simulink model "EvPowertrainController3EMDualRear"  (R2024a)
settings: configuration reference "VehicleFixed10ms" (kept outside this file)
model workspace (MAT data in the model file):
  CtrlVcuAccelPdlBpts = [0 0.8 1]
  CtrlVcuBattPnlty = 10000000
  CtrlVcuBattSOCBpts = [0 20 60 80 100]
  CtrlVcuCnstrntPnltyFctr = 10000000
  CtrlVcuEMPnlty = 100
  CtrlVcuEMTrqSplitGrid = 200
  CtrlVcuFallRate = -500
  CtrlVcuMaxAccelG = 1
  CtrlVcuMaxDecelG = -1.5
  CtrlVcuPwrDeltaPnlty = 50
  CtrlVcuPwrRatePnlty = [25 25 100]
  CtrlVcuRiseRate = 500
  CtrlVcuRoadMuEst = 0.8
  CtrlVcuSftyFctr = 0.9
  CtrlVcuTracPwrErrPnlty = 25
  CtrlVcuTrqVecBrkThresh = 0.01
  CtrlVcuTrqVecIGain = 0
  CtrlVcuTrqVecMinTrq = 25
  CtrlVcuTrqVecPGain = -2000
  CtrlVcuTrqVecSteerThresh = 0.349065850399
  CtrlVcuTrqVecVelThresh = 2.5
  N_P0 = 3
undefined symbols (not defined in the file): CtrlBcuTrlrBrkGain, CtrlVcuEvChrgLmtBpt, CtrlVcuEvRegenBrkCutOff, CtrlVcuEvRegenBrkSpdBpt, CtrlVcuEvSocBpt, eff, EnvGrvty, PlntBrkActrBoreFrnt, PlntBrkFrntBias, PlntBrkKinFricCffFrnt, PlntBrkNumPadsFrnt, PlntBrkPadMeanRadiusFrnt, PlntBrkPrsFctr, PlntBrkRearBias, PlntDiffrntl2Eff, PlntDiffrntl2Ratio, PlntDiffrntlEff, PlntDiffrntlRatio, PlntEM1EffTbl, PlntEM1Spd, PlntEM1SpdEff, PlntEM1Trq, PlntEM1TrqEff, PlntEM2EffTbl, PlntEM2Spd, PlntEM2SpdEff, PlntEM2Trq, PlntEM2TrqEff, PlntEM3EffTbl, PlntEM3Spd, PlntEM3SpdEff, PlntEM3Trq, PlntEM3TrqEff, PlntEMWhlGearEffFL, PlntEMWhlGearEffRL, PlntEMWhlGearRatioFL, PlntEMWhlGearRatioRL, PlntTransEffSpdBpt, PlntTransEffTbl, PlntTransEffTempBpt, PlntTransEffTrqBpt, PlntTransGearNumVect, PlntTransGearRatioVect, PlntVehCGHgtAxl, PlntVehDstCGFrntAxl, PlntVehDstCGRearAxl, PlntVehMass, PlntWhlLdRadius
libraries: simulink x16, autolibutils x2, slpidlib x2
(part 1 of 5)
settings Model: DataDictionary=VirtualVehicleTemplate.sldd  ModifiedByFormat=The MathWorks, Inc.  Creator=The MathWorks, Inc.  LastModifiedBy=The MathWorks, Inc.
settings ConfigSetRef: SourceName=VehicleFixed10ms

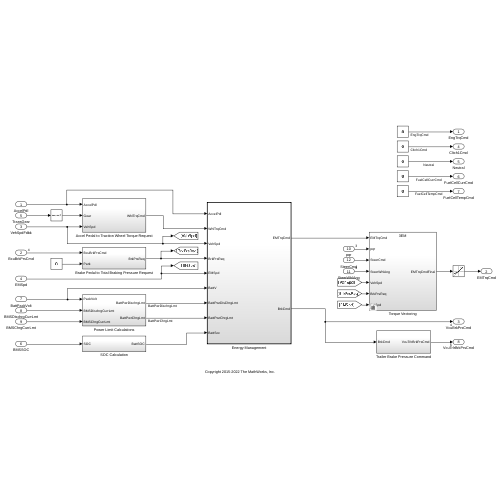
[thumbnail: Simulink's stored preview of the top-level diagram]
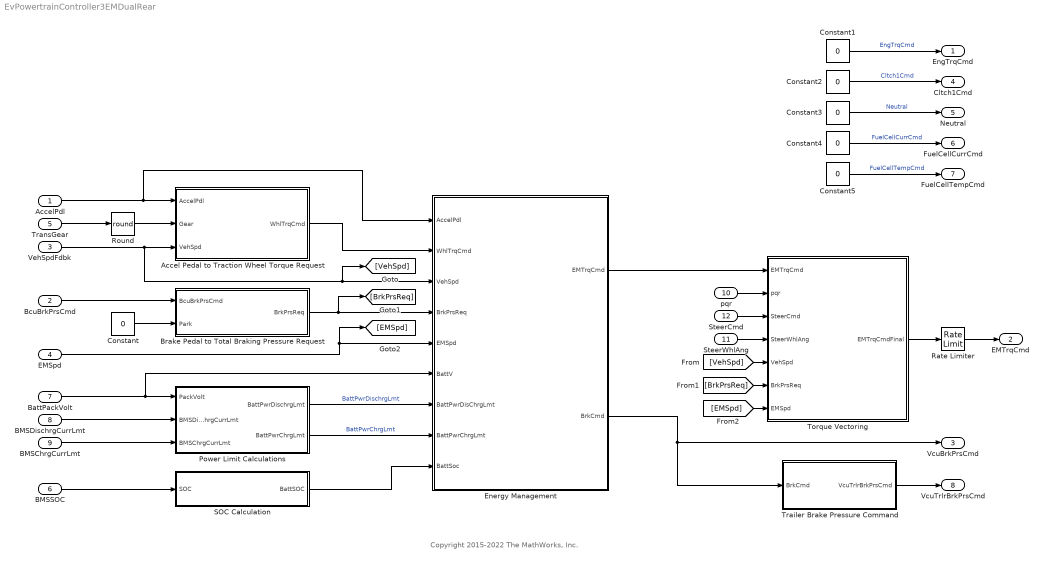
== system EvPowertrainController3EMDualRear ==
  note: Copyright 2015-2022 The MathWorks, Inc.
  AccelPdl : Inport  OutDataTypeStr=double  PortDimensions=1
  BcuBrkPrsCmd : Inport  Port=2  OutDataTypeStr=double  PortDimensions=4
  VehSpdFdbk : Inport  Port=3  OutDataTypeStr=double  PortDimensions=1
  EMSpd : Inport  Port=4  OutDataTypeStr=double
  TransGear : Inport  Port=5  OutDataTypeStr=double  PortDimensions=1
  BMSSOC : Inport  Port=6
  BattPackVolt : Inport  Port=7
  BMSDischrgCurrLmt : Inport  Port=8
  BMSChrgCurrLmt : Inport  Port=9
  pqr : Inport  Port=10  PortDimensions=3
  SteerWhlAng : Inport  Port=11  PortDimensions=4
  SteerCmd : Inport  Port=12
  Accel Pedal to Traction Wheel Torque Request : Subsystem  InitFcn=[~]=autosharedicon('autolibinternalvvblock',gcb,0);  VariantControl=Choice
  Brake Pedal to Total Braking Pressure Request : Subsystem  InitFcn=[~]=autosharedicon('autolibinternalvvblock',gcb,0);
  Constant{,1..5} (6 alike) : Constant  Value=0  SampleTime=-1
  Energy Management : Subsystem  LoadFcn=[~]=autosharedicon('autolibinternalvvblock',gcb,0);  TreatAsAtomicUnit=on
  Power Limit Calculations : Subsystem  InitFcn=[~]=autosharedicon('autolibinternalvvblock',gcb,0);
  Rate Limiter : RateLimiter  RisingSlewLimit=CtrlVcuRiseRate  FallingSlewLimit=CtrlVcuFallRate  SampleTimeMode=inherited
  Round : Rounding  Operator=round
  SOC Calculation : Subsystem  InitFcn=[~]=autosharedicon('autolibinternalvvblock',gcb,0);
  Torque Vectoring : Subsystem  Variant=on  VariantControlMode=label  VariantControl=Choice  LabelModeActiveChoice=3EM
  Trailer Brake Pressure Command : Subsystem
  EngTrqCmd : Outport  OutDataTypeStr=double  PortDimensions=1  VectorParamsAs1DForOutWhenUnconnected=off
  EMTrqCmd : Outport  Port=2  OutDataTypeStr=double  VectorParamsAs1DForOutWhenUnconnected=off
  VcuBrkPrsCmd : Outport  Port=3  OutDataTypeStr=double  PortDimensions=4  VectorParamsAs1DForOutWhenUnconnected=off
  Cltch1Cmd : Outport  Port=4  OutDataTypeStr=double  PortDimensions=1  VectorParamsAs1DForOutWhenUnconnected=off
  Neutral : Outport  Port=5  OutDataTypeStr=double  PortDimensions=1  VectorParamsAs1DForOutWhenUnconnected=off
  FuelCellCurrCmd : Outport  Port=6  OutDataTypeStr=double  PortDimensions=1
  FuelCellTempCmd : Outport  Port=7  OutDataTypeStr=double  PortDimensions=1
  VcuTrlrBrkPrsCmd : Outport  Port=8  PortDimensions=6  VectorParamsAs1DForOutWhenUnconnected=off
  wires:
  AccelPdl/1 -> Energy Management/1(AccelPdl), Accel Pedal to Traction Wheel Torque Request/1(AccelPdl)
  BcuBrkPrsCmd/1 -> Brake Pedal to Total Braking Pressure Request/1(BcuBrkPrsCmd)
  Constant/1 -> Brake Pedal to Total Braking Pressure Request/2(Park)
  Brake Pedal to Total Braking Pressure Request/1(BrkPrsReq) -> [BrkPrsReq], Energy Management/4("BrkPrsReq ")
  VehSpdFdbk/1 -> [VehSpd], Energy Management/3(VehSpd), Accel Pedal to Traction Wheel Torque Request/3(VehSpd)
  Constant2/1 -> Cltch1Cmd/1  "Cltch1Cmd"
  Constant3/1 -> Neutral/1  "Neutral"
  Constant1/1 -> EngTrqCmd/1  "EngTrqCmd"
  Constant4/1 -> FuelCellCurrCmd/1  "FuelCellCurrCmd"
  Constant5/1 -> FuelCellTempCmd/1  "FuelCellTempCmd"
  Accel Pedal to Traction Wheel Torque Request/1(WhlTrqCmd) -> Energy Management/2(WhlTrqCmd)
  TransGear/1 -> Round/1
  Round/1 -> Accel Pedal to Traction Wheel Torque Request/2(Gear)
  BMSChrgCurrLmt/1 -> Power Limit Calculations/3(BMSChrgCurrLmt)
  BMSSOC/1 -> SOC Calculation/1(SOC)
  BattPackVolt/1 -> Energy Management/6(BattV), Power Limit Calculations/1(PackVolt)
  BMSDischrgCurrLmt/1 -> Power Limit Calculations/2(BMSDischrgCurrLmt)
  Power Limit Calculations/1(BattPwrDischrgLmt) -> Energy Management/7(BattPwrDisChrgLmt)  "BattPwrDischrgLmt"
  Power Limit Calculations/2(BattPwrChrgLmt) -> Energy Management/8("BattPwrChrgLmt ")  "BattPwrChrgLmt"
  SOC Calculation/1(BattSOC) -> Energy Management/9(BattSoc)
  EMSpd/1 -> [EMSpd], Energy Management/5(EMSpd)
  Energy Management/1(EMTrqCmd) -> Torque Vectoring/1(EMTrqCmd)
  pqr/1 -> Torque Vectoring/2(pqr)
  SteerCmd/1 -> Torque Vectoring/3(SteerCmd)
  SteerWhlAng/1 -> Torque Vectoring/4(SteerWhlAng)
  [VehSpd] -> Torque Vectoring/5(VehSpd)
  [BrkPrsReq] -> Torque Vectoring/6(BrkPrsReq)
  [EMSpd] -> Torque Vectoring/7(EMSpd)
  Torque Vectoring/1(EMTrqCmdFinal) -> Rate Limiter/1
  Rate Limiter/1 -> EMTrqCmd/1
  Energy Management/2(BrkCmd) -> Trailer Brake Pressure Command/1(BrkCmd), VcuBrkPrsCmd/1
  Trailer Brake Pressure Command/1(VcuTrlrBrkPrsCmd) -> VcuTrlrBrkPrsCmd/1

== system EvPowertrainController3EMDualRear/Accel Pedal to Traction Wheel Torque Request ==
  note: Convert Accelerator Pedal Position to
      | Wheel Torque Command using Motor
      | Torque Speed Curves.
      |
      | Can be replaced with 2D Lookup Table
      | with AccelPdl and VehSpd as inputs and
      | Motor or Wheel Torque Command as output.
  AccelPdl : Inport
  Gear : Inport  Port=2
  VehSpd : Inport  Port=3
  EM2WhlTrq : Subsystem  Variant=on  VariantControlMode=label  VariantControl=Choice  LabelModeActiveChoice=3EM Dual Rear
  Product1 : Product
  WhlTrqCmd : Outport  VectorParamsAs1DForOutWhenUnconnected=off
  wires:
  Product1/1 -> WhlTrqCmd/1
  AccelPdl/1 -> Product1/1
  Gear/1 -> EM2WhlTrq/1(Gear)
  VehSpd/1 -> EM2WhlTrq/2(VehSpd)
  EM2WhlTrq/1(WhlTrqCmd) -> Product1/2

== system EvPowertrainController3EMDualRear/Brake Pedal to Total Braking Pressure Request ==
  BcuBrkPrsCmd : Inport
  Park : Inport  Port=2
  Front Bias : Constant  Value=PlntBrkFrntBias
  Gain4 : Gain  Gain=PlntBrkPrsFctr
  Mux : Mux
  Product : Product
  Rear Bias : Constant  Value=PlntBrkRearBias
  Terminator : Terminator
  BrkPrsReq : Outport  VectorParamsAs1DForOutWhenUnconnected=off
  wires:
  BcuBrkPrsCmd/1 -> Product/2
  Mux/1 -> Product/1
  Rear Bias/1 -> Mux/4, Mux/3
  Front Bias/1 -> Mux/1, Mux/2
  Gain4/1 -> BrkPrsReq/1
  Product/1 -> Gain4/1
  Park/1 -> Terminator/1

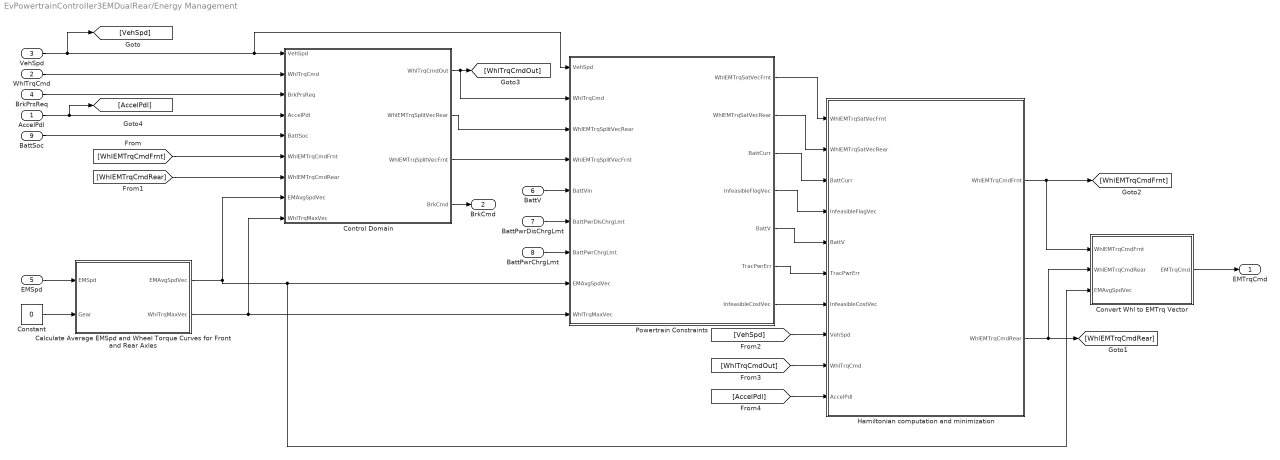
== system EvPowertrainController3EMDualRear/Energy Management ==
  AccelPdl : Inport
  WhlTrqCmd : Inport  Port=2
  VehSpd : Inport  Port=3
  "BrkPrsReq " : Inport  Port=4
  EMSpd : Inport  Port=5
  BattV : Inport  Port=6
  BattPwrDisChrgLmt : Inport  Port=7
  "BattPwrChrgLmt " : Inport  Port=8
  BattSoc : Inport  Port=9
  Calculate Average EMSpd and Wheel Torque Curves for Front and Rear Axles : Subsystem  Variant=on  VariantControlMode=label  VariantControl=Choice  LabelModeActiveChoice=3EM Dual Rear
  Constant : Constant  Value=0  SampleTime=-1
  "Control Domain " : Subsystem  InitFcn="[~] =  autosharedeval('1');"
  Convert Whl to EMTrq Vector : Subsystem  Variant=on  VariantControlMode=label  VariantControl=Choice  LabelModeActiveChoice=3EM Dual Rear
  Hamiltonian computation and minimization : Subsystem  InitFcn="[~] =  autosharedeval('1');"
  "Powertrain Constraints " : Subsystem  InitFcn="[~] =  autosharedeval('1');"
  EMTrqCmd : Outport  VectorParamsAs1DForOutWhenUnconnected=off
  BrkCmd : Outport  Port=2  VectorParamsAs1DForOutWhenUnconnected=off
  wires:
  "Control Domain "/1(WhlTrqCmdOut) -> "Powertrain Constraints "/2(WhlTrqCmd), [WhlTrqCmdOut]
  "BrkPrsReq "/1 -> "Control Domain "/3("BrkPrsReq ")
  AccelPdl/1 -> [AccelPdl], "Control Domain "/4(AccelPdl)
  "Control Domain "/4(BrkCmd) -> BrkCmd/1
  "Powertrain Constraints "/6(TracPwrErr) -> Hamiltonian computation and minimization/6(TracPwrErr)
  BattV/1 -> "Powertrain Constraints "/5(BattVin)
  VehSpd/1 -> [VehSpd], "Control Domain "/1(VehSpd), "Powertrain Constraints "/1(VehSpd)
  Hamiltonian computation and minimization/2(WhlEMTrqCmdRear) -> Convert Whl to EMTrq Vector/2(WhlEMTrqCmdRear), [WhlEMTrqCmdRear]
  Hamiltonian computation and minimization/1(WhlEMTrqCmdFrnt) -> [WhlEMTrqCmdFrnt], Convert Whl to EMTrq Vector/1(WhlEMTrqCmdFrnt)
  "Powertrain Constraints "/4(InfeasibleFlagVec) -> Hamiltonian computation and minimization/4(InfeasibleFlagVec)
  "Powertrain Constraints "/3(BattCurr) -> Hamiltonian computation and minimization/3(BattCurr)
  "Powertrain Constraints "/5(BattV) -> Hamiltonian computation and minimization/5(BattV)
  WhlTrqCmd/1 -> "Control Domain "/2(WhlTrqCmd)
  "Control Domain "/2(WhlEMTrqSplitVecRear) -> "Powertrain Constraints "/3(WhlEMTrqSplitVecRear)
  Calculate Average EMSpd and Wheel Torque Curves for Front and Rear Axles/1(EMAvgSpdVec) -> "Control Domain "/8(EMAvgSpdVec), Convert Whl to EMTrq Vector/3(EMAvgSpdVec), "Powertrain Constraints "/8(EMAvgSpdVec)
  "BattPwrChrgLmt "/1 -> "Powertrain Constraints "/7("BattPwrChrgLmt ")
  BattPwrDisChrgLmt/1 -> "Powertrain Constraints "/6(BattPwrDisChrgLmt)
  [WhlEMTrqCmdFrnt] -> "Control Domain "/6(WhlEMTrqCmdFrnt)
  BattSoc/1 -> "Control Domain "/5(BattSoc)
  EMSpd/1 -> Calculate Average EMSpd and Wheel Torque Curves for Front and Rear Axles/1(EMSpd)
  Convert Whl to EMTrq Vector/1(EMTrqCmd) -> EMTrqCmd/1
  [WhlEMTrqCmdRear] -> "Control Domain "/7(WhlEMTrqCmdRear)
  Constant/1 -> Calculate Average EMSpd and Wheel Torque Curves for Front and Rear Axles/2(Gear)
  Calculate Average EMSpd and Wheel Torque Curves for Front and Rear Axles/2(WhlTrqMaxVec) -> "Control Domain "/9(WhlTrqMaxVec), "Powertrain Constraints "/9(WhlTrqMaxVec)
  "Powertrain Constraints "/1(WhlEMTrqSatVecFrnt) -> Hamiltonian computation and minimization/1(WhlEMTrqSatVecFrnt)
  "Powertrain Constraints "/2(WhlEMTrqSatVecRear) -> Hamiltonian computation and minimization/2(WhlEMTrqSatVecRear)
  [VehSpd] -> Hamiltonian computation and minimization/8(VehSpd)
  "Powertrain Constraints "/7(InfeasibleCostVec) -> Hamiltonian computation and minimization/7(InfeasibleCostVec)
  "Control Domain "/3(WhlEMTrqSplitVecFrnt) -> "Powertrain Constraints "/4(WhlEMTrqSplitVecFrnt)
  [WhlTrqCmdOut] -> Hamiltonian computation and minimization/9(WhlTrqCmd)
  [AccelPdl] -> Hamiltonian computation and minimization/10(AccelPdl)

== system EvPowertrainController3EMDualRear/Power Limit Calculations ==
  note: BMS has opposite sign convention for current
  note: Use Current Limits from BMS to calculate
      | discharge and charge power limits
  PackVolt : Inport
  BMSDischrgCurrLmt : Inport  Port=2
  BMSChrgCurrLmt : Inport  Port=3
  Data Type Conversion : DataTypeConversion  SaturateOnIntegerOverflow=off  RndMeth=Floor
  Data Type Conversion1 : DataTypeConversion  SaturateOnIntegerOverflow=off  RndMeth=Floor
  Gain : Gain  Gain=-1
  Gain1 : Gain  Gain=-1
  Product : Product
  Product1 : Product
  BattPwrDischrgLmt : Outport  VectorParamsAs1DForOutWhenUnconnected=off
  BattPwrChrgLmt : Outport  Port=2  VectorParamsAs1DForOutWhenUnconnected=off
  wires:
  Gain/1 -> Product1/2
  Gain1/1 -> Product/2
  Product/1 -> Data Type Conversion1/1
  Product1/1 -> Data Type Conversion/1
  PackVolt/1 -> Product/1, Product1/1
  BMSChrgCurrLmt/1 -> Gain/1
  BMSDischrgCurrLmt/1 -> Gain1/1
  Data Type Conversion/1 -> BattPwrChrgLmt/1
  Data Type Conversion1/1 -> BattPwrDischrgLmt/1

== system EvPowertrainController3EMDualRear/SOC Calculation ==
  SOC : Inport
  Data Type Conversion : DataTypeConversion  SaturateOnIntegerOverflow=off  RndMeth=Floor
  convert2percent : Gain  Gain=100
  BattSOC : Outport
  wires:
  convert2percent/1 -> Data Type Conversion/1
  SOC/1 -> convert2percent/1
  Data Type Conversion/1 -> BattSOC/1

== system EvPowertrainController3EMDualRear/Torque Vectoring ==
  EMTrqCmd : Inport
  pqr : Inport  Port=2
  SteerCmd : Inport  Port=3
  SteerWhlAng : Inport  Port=4
  VehSpd : Inport  Port=5
  BrkPrsReq : Inport  Port=6
  EMSpd : Inport  Port=7
  3EM : Subsystem  LoadFcn=[~]=autosharedicon('autolibinternalvvblock',gcb,0);  VariantControl=3EM
  4EM : Subsystem  LoadFcn=[~]=autosharedicon('autolibinternalvvblock',gcb,0);  VariantControl=4EM
  No Torque Vectoring : Subsystem  VariantControl=No Torque Vectoring
  EMTrqCmdFinal : Outport

== system EvPowertrainController3EMDualRear/Trailer Brake Pressure Command ==
  BrkCmd : Inport
  Gain1 : Gain  Gain=CtrlBcuTrlrBrkGain
  Probe : Probe  ProbeSampleTime=off  ProbeComplexSignal=off
  Product : Product  Inputs=*/
  Selector2 : Selector  InputPortWidth=1  IndexOptions=Index vector (dialog)  Indices=[1 1 1 1 1 1]  OutputSizes=1
  Sum : Sum  Inputs=+
  VcuTrlrBrkPrsCmd : Outport
  wires:
  Gain1/1 -> Selector2/1
  Product/1 -> Gain1/1
  Probe/1 -> Product/2
  BrkCmd/1 -> Probe/1, Sum/1
  Sum/1 -> Product/1
  Selector2/1 -> VcuTrlrBrkPrsCmd/1

== system EvPowertrainController3EMDualRear/Accel Pedal to Traction Wheel Torque Request/EM2WhlTrq ==
  Gear : Inport
  VehSpd : Inport  Port=2
  2EM : Subsystem  VariantControl=2EM
  3EM Dual Front : Subsystem  VariantControl=3EM Dual Front
  3EM Dual Rear : Subsystem  VariantControl=3EM Dual Rear
  4EM : Subsystem  VariantControl=4EM
  WhlTrqCmd : Outport

== system EvPowertrainController3EMDualRear/Energy Management/Calculate Average EMSpd and Wheel Torque Curves for Front and Rear Axles ==
  EMSpd : Inport
  Gear : Inport  Port=2
  2EM : Subsystem  VariantControl=2EM
  3EM Dual Front : Subsystem  VariantControl=3EM Dual Front
  3EM Dual Rear : Subsystem  VariantControl=3EM Dual Rear
  4EM : Subsystem  VariantControl=4EM
  EMAvgSpdVec : Outport
  WhlTrqMaxVec : Outport  Port=2

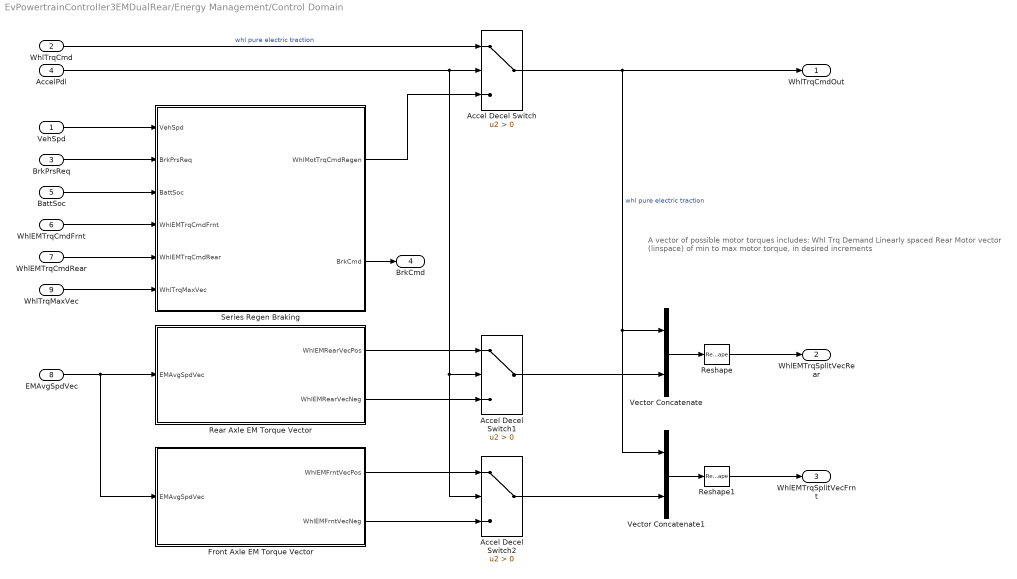
== system EvPowertrainController3EMDualRear/Energy Management/Control Domain  ==
  note: A vector of possible motor torques includes:
      | Whl Trq Demand
      | Linearly spaced Rear Motor vector (linspace) of min to max motor torque, in desired increments
  VehSpd : Inport
  WhlTrqCmd : Inport  Port=2
  "BrkPrsReq " : Inport  Port=3
  AccelPdl : Inport  Port=4
  BattSoc : Inport  Port=5
  WhlEMTrqCmdFrnt : Inport  Port=6
  WhlEMTrqCmdRear : Inport  Port=7
  EMAvgSpdVec : Inport  Port=8
  WhlTrqMaxVec : Inport  Port=9
  Accel Decel Switch : Switch  Criteria=u2 > Threshold  SaturateOnIntegerOverflow=off  InputSameDT=off
  Accel Decel Switch1 : Switch  Criteria=u2 > Threshold  SaturateOnIntegerOverflow=off  InputSameDT=off
  Accel Decel Switch2 : Switch  Criteria=u2 > Threshold  SaturateOnIntegerOverflow=off  InputSameDT=off
  Front Axle EM Torque Vector : Subsystem  Variant=on  VariantControlMode=label  VariantControl=Choice  LabelModeActiveChoice=2EM or 3EM Dual Rear
  Rear Axle EM Torque Vector : Subsystem  Variant=on  VariantControlMode=label  VariantControl=Choice  LabelModeActiveChoice=3EM Dual Rear or 4EM
  Reshape : Reshape
  Reshape1 : Reshape
  Series Regen Braking : Subsystem  InitFcn=%[~]=autosharedicon('autolibutils',gcb,0);  VariantControl=Variant
  Vector Concatenate : Concatenate
  Vector Concatenate1 : Concatenate
  WhlTrqCmdOut : Outport  VectorParamsAs1DForOutWhenUnconnected=off
  WhlEMTrqSplitVecRear : Outport  Port=2  VectorParamsAs1DForOutWhenUnconnected=off
  WhlEMTrqSplitVecFrnt : Outport  Port=3  VectorParamsAs1DForOutWhenUnconnected=off
  BrkCmd : Outport  Port=4  VectorParamsAs1DForOutWhenUnconnected=off
  wires:
  Vector Concatenate/1 -> Reshape/1
  Reshape/1 -> WhlEMTrqSplitVecRear/1
  WhlTrqMaxVec/1 -> Series Regen Braking/6(WhlTrqMaxVec)
  AccelPdl/1 -> Accel Decel Switch2/2, Accel Decel Switch1/2, Accel Decel Switch/2
  Series Regen Braking/2(" BrkCmd") -> BrkCmd/1
  WhlTrqCmd/1 -> Accel Decel Switch/1  "whl pure electric traction"
  "BrkPrsReq "/1 -> Series Regen Braking/2("BrkPrsReq ")
  EMAvgSpdVec/1 -> Front Axle EM Torque Vector/1(EMAvgSpdVec), Rear Axle EM Torque Vector/1(EMAvgSpdVec)
  VehSpd/1 -> Series Regen Braking/1(VehSpd)
  Accel Decel Switch/1 -> Vector Concatenate/1, Vector Concatenate1/1, WhlTrqCmdOut/1  "whl pure electric traction"
  Accel Decel Switch1/1 -> Vector Concatenate/2
  Series Regen Braking/1(" WhlMotTrqCmdRegen") -> Accel Decel Switch/3
  WhlEMTrqCmdFrnt/1 -> Series Regen Braking/4(WhlEMTrqCmdFrnt)
  WhlEMTrqCmdRear/1 -> Series Regen Braking/5(WhlEMTrqCmdRear)
  BattSoc/1 -> Series Regen Braking/3(BattSoc)
  Rear Axle EM Torque Vector/1(WhlEMRearVecPos) -> Accel Decel Switch1/1
  Rear Axle EM Torque Vector/2(WhlEMRearVecNeg) -> Accel Decel Switch1/3
  Reshape1/1 -> WhlEMTrqSplitVecFrnt/1
  Vector Concatenate1/1 -> Reshape1/1
  Front Axle EM Torque Vector/1(WhlEMFrntVecPos) -> Accel Decel Switch2/1
  Front Axle EM Torque Vector/2(WhlEMFrntVecNeg) -> Accel Decel Switch2/3
  Accel Decel Switch2/1 -> Vector Concatenate1/2

== system EvPowertrainController3EMDualRear/Energy Management/Convert Whl to EMTrq Vector ==
  WhlEMTrqCmdFrnt : Inport
  WhlEMTrqCmdRear : Inport  Port=2
  EMAvgSpdVec : Inport  Port=3
  2EM : Subsystem  VariantControl=2EM
  3EM Dual Front : Subsystem  VariantControl=3EM Dual Front
  3EM Dual Rear : Subsystem  VariantControl=3EM Dual Rear
  4EM : Subsystem  VariantControl=4EM
  EMTrqCmd : Outport

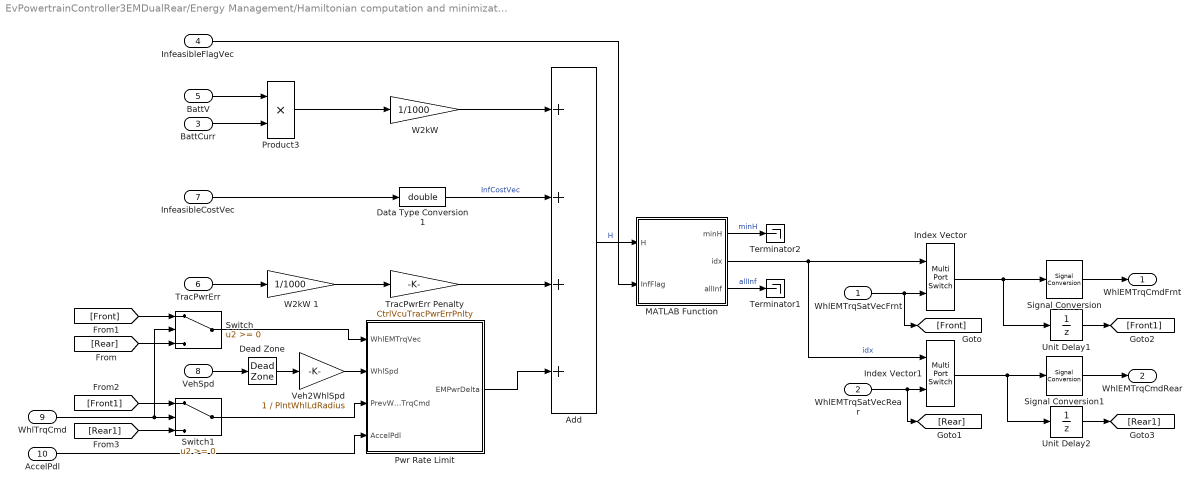
== system EvPowertrainController3EMDualRear/Energy Management/Hamiltonian computation and minimization ==
  WhlEMTrqSatVecFrnt : Inport
  WhlEMTrqSatVecRear : Inport  Port=2
  BattCurr : Inport  Port=3
  InfeasibleFlagVec : Inport  Port=4
  BattV : Inport  Port=5
  TracPwrErr : Inport  Port=6
  InfeasibleCostVec : Inport  Port=7
  VehSpd : Inport  Port=8
  WhlTrqCmd : Inport  Port=9
  AccelPdl : Inport  Port=10
  Add : Sum  Inputs=++++
  Data Type Conversion1 : DataTypeConversion  OutDataTypeStr=double  SaturateOnIntegerOverflow=off  RndMeth=Floor
  Dead Zone : DeadZone  LowerValue=-0.1  UpperValue=0.1
  Index Vector : MultiPortSwitch  Inputs=1  SaturateOnIntegerOverflow=off  InputSameDT=off
  Index Vector1 : MultiPortSwitch  Inputs=1  SaturateOnIntegerOverflow=off  InputSameDT=off
  MATLAB Function : MATLAB Function  InitFcn="[~] =  autosharedeval('1');"  TreatAsAtomicUnit=on
  Product3 : Product
  Pwr Rate Limit : Subsystem  InitFcn="[~] =  autosharedeval('1');"
  Signal Conversion : SignalConversion  OverrideOpt=off
  Signal Conversion1 : SignalConversion  OverrideOpt=off
  Switch : Switch  SaturateOnIntegerOverflow=off  InputSameDT=off
  Switch1 : Switch  SaturateOnIntegerOverflow=off  InputSameDT=off
  Terminator1 : Terminator
  Terminator2 : Terminator
  TracPwrErr Penalty : Gain  Gain=CtrlVcuTracPwrErrPnlty
  Unit Delay1 : UnitDelay  SampleTime=-1  HasFrameUpgradeWarning=on
  Unit Delay2 : UnitDelay  SampleTime=-1  HasFrameUpgradeWarning=on
  Veh2WhlSpd : Gain  Gain=1 / PlntWhlLdRadius
  "W2kW " : Gain  Gain=1/1000
  W2kW 1 : Gain  Gain=1/1000
  WhlEMTrqCmdFrnt : Outport  VectorParamsAs1DForOutWhenUnconnected=off
  WhlEMTrqCmdRear : Outport  Port=2  VectorParamsAs1DForOutWhenUnconnected=off
  wires:
  Data Type Conversion1/1 -> Add/2  "InfCostVec"
  TracPwrErr Penalty/1 -> Add/3
  W2kW 1/1 -> TracPwrErr Penalty/1
  TracPwrErr/1 -> W2kW 1/1
  Signal Conversion1/1 -> WhlEMTrqCmdRear/1
  Signal Conversion/1 -> WhlEMTrqCmdFrnt/1
  Index Vector/1 -> Unit Delay1/1, Signal Conversion/1
  "W2kW "/1 -> Add/1
  BattV/1 -> Product3/1
  Index Vector1/1 -> Unit Delay2/1, Signal Conversion1/1
  Add/1 -> MATLAB Function/1(H)  "H"
  MATLAB Function/1(minH) -> Terminator2/1  "minH"
  MATLAB Function/2(idx) -> Index Vector1/1, Index Vector/1  "idx"
  WhlEMTrqSatVecRear/1 -> [Rear], Index Vector1/2
  InfeasibleFlagVec/1 -> MATLAB Function/2(InfFlag)
  WhlEMTrqSatVecFrnt/1 -> [Front], Index Vector/2
  Product3/1 -> "W2kW "/1
  [Front] -> Switch/1
  Veh2WhlSpd/1 -> Pwr Rate Limit/2(WhlSpd)
  MATLAB Function/3(allInf) -> Terminator1/1  "allInf"
  Pwr Rate Limit/1(EMPwrDelta) -> Add/4
  VehSpd/1 -> Dead Zone/1
  InfeasibleCostVec/1 -> Data Type Conversion1/1
  [Rear] -> Switch/3
  [Front1] -> Switch1/1
  BattCurr/1 -> Product3/2
  WhlTrqCmd/1 -> Switch/2, Switch1/2
  Unit Delay1/1 -> [Front1]
  Unit Delay2/1 -> [Rear1]
  [Rear1] -> Switch1/3
  Dead Zone/1 -> Veh2WhlSpd/1
  Switch/1 -> Pwr Rate Limit/1(WhlEMTrqVec)
  Switch1/1 -> Pwr Rate Limit/3(PrevWhlEMTrqCmd)
  AccelPdl/1 -> Pwr Rate Limit/4(AccelPdl)

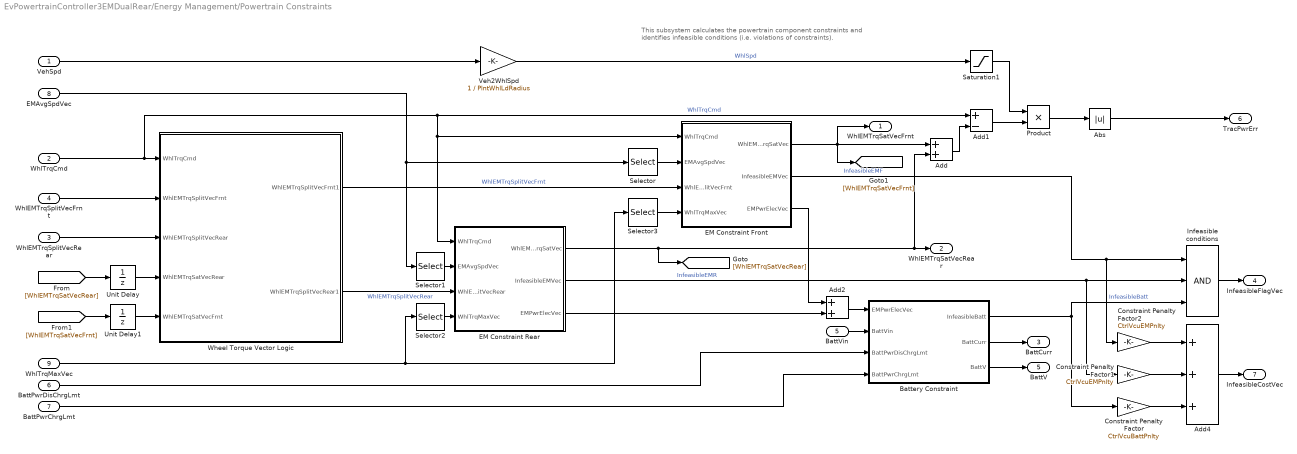
== system EvPowertrainController3EMDualRear/Energy Management/Powertrain Constraints  ==
  note: This subsystem calculates the powertrain component constraints
      | and identifies infeasible conditions (i.e. violations of constraints).
  VehSpd : Inport
  WhlTrqCmd : Inport  Port=2
  WhlEMTrqSplitVecRear : Inport  Port=3
  WhlEMTrqSplitVecFrnt : Inport  Port=4
  BattVin : Inport  Port=5
  BattPwrDisChrgLmt : Inport  Port=6
  "BattPwrChrgLmt " : Inport  Port=7
  EMAvgSpdVec : Inport  Port=8
  WhlTrqMaxVec : Inport  Port=9
  Abs : Abs  SaturateOnIntegerOverflow=off
  Add : Sum
  Add1 : Sum  Inputs=+-
  Add2 : Sum
  Add4 : Sum  Inputs=+++
  Battery Constraint : Subsystem  InitFcn="[~] =  autosharedeval('1');"
  Constraint Penalty Factor : Gain  Gain=CtrlVcuBattPnlty
  Constraint Penalty Factor1 : Gain  Gain=CtrlVcuEMPnlty
  Constraint Penalty Factor2 : Gain  Gain=CtrlVcuEMPnlty
  EM Constraint Front : Subsystem  InitFcn="[~] =  autosharedeval('1');"
  EM Constraint Rear : Subsystem  InitFcn="[~] =  autosharedeval('1');"
  Infeasible conditions : Logic  Inputs=3  AllPortsSameDT=off  OutDataTypeStr=boolean
  Product : Product
  Saturation1 : Saturate  UpperLimit=inf  LowerLimit=0.001
  Selector : Selector  InputPortWidth=2  IndexOptions=Index vector (dialog)  Indices=[1]  OutputSizes=1
  Selector1 : Selector  InputPortWidth=2  IndexOptions=Index vector (dialog)  Indices=[2]  OutputSizes=1
  Selector2 : Selector  InputPortWidth=2  IndexOptions=Index vector (dialog)  Indices=[2]  OutputSizes=1
  Selector3 : Selector  InputPortWidth=2  IndexOptions=Index vector (dialog)  Indices=[1]  OutputSizes=1
  Unit Delay : UnitDelay  SampleTime=-1  HasFrameUpgradeWarning=on
  Unit Delay1 : UnitDelay  SampleTime=-1  HasFrameUpgradeWarning=on
  Veh2WhlSpd : Gain  Gain=1 / PlntWhlLdRadius
  Wheel Torque Vector Logic : Subsystem
  WhlEMTrqSatVecFrnt : Outport  VectorParamsAs1DForOutWhenUnconnected=off
  WhlEMTrqSatVecRear : Outport  Port=2  VectorParamsAs1DForOutWhenUnconnected=off
  BattCurr : Outport  Port=3  VectorParamsAs1DForOutWhenUnconnected=off
  InfeasibleFlagVec : Outport  Port=4  VectorParamsAs1DForOutWhenUnconnected=off
  BattV : Outport  Port=5  VectorParamsAs1DForOutWhenUnconnected=off
  TracPwrErr : Outport  Port=6  VectorParamsAs1DForOutWhenUnconnected=off
  InfeasibleCostVec : Outport  Port=7  VectorParamsAs1DForOutWhenUnconnected=off
  wires:
  EM Constraint Rear/1(WhlEMTrqSatVec) -> WhlEMTrqSatVecRear/1, Add/2, [WhlEMTrqSatVecRear]
  Add/1 -> Add1/2
  Add1/1 -> Product/2
  Battery Constraint/1(InfeasibleBatt) -> Constraint Penalty Factor/1, Infeasible conditions/3  "InfeasibleBatt"
  Infeasible conditions/1 -> InfeasibleFlagVec/1
  EM Constraint Rear/2(InfeasibleEMVec) -> Constraint Penalty Factor1/1, Infeasible conditions/2  "InfeasibleEMR"
  Abs/1 -> TracPwrErr/1
  Veh2WhlSpd/1 -> Saturation1/1  "WhlSpd"
  Saturation1/1 -> Product/1
  BattVin/1 -> Battery Constraint/2(BattVin)
  WhlTrqCmd/1 -> EM Constraint Front/1(WhlTrqCmd), EM Constraint Rear/1(WhlTrqCmd), Add1/1, Wheel Torque Vector Logic/1(WhlTrqCmd)  "WhlTrqCmd"
  EM Constraint Front/1(WhlEMTrqSatVec) -> WhlEMTrqSatVecFrnt/1, [WhlEMTrqSatVecFrnt], Add/1
  Battery Constraint/2(BattCurr) -> BattCurr/1
  EM Constraint Front/2(InfeasibleEMVec) -> Constraint Penalty Factor2/1, Infeasible conditions/1  "InfeasibleEMF"
  Add2/1 -> Battery Constraint/1(EMPwrElecVec)
  EM Constraint Rear/3(EMPwrElecVec) -> Add2/2
  Battery Constraint/3(BattV) -> BattV/1
  EMAvgSpdVec/1 -> Selector/1, Selector1/1
  Wheel Torque Vector Logic/1(WhlEMTrqSplitVecFrnt1) -> EM Constraint Front/3(WhlEMTrqSplitVecFrnt)  "WhlEMTrqSplitVecFrnt"
  Product/1 -> Abs/1
  EM Constraint Front/3(EMPwrElecVec) -> Add2/1
  Selector/1 -> EM Constraint Front/2(EMAvgSpdVec)
  Selector1/1 -> EM Constraint Rear/2(EMAvgSpdVec)
  Selector2/1 -> EM Constraint Rear/4(WhlTrqMaxVec)
  Selector3/1 -> EM Constraint Front/4(WhlTrqMaxVec)
  Add4/1 -> InfeasibleCostVec/1
  Constraint Penalty Factor/1 -> Add4/3
  Constraint Penalty Factor1/1 -> Add4/2
  Constraint Penalty Factor2/1 -> Add4/1
  BattPwrDisChrgLmt/1 -> Battery Constraint/3(BattPwrDisChrgLmt)
  "BattPwrChrgLmt "/1 -> Battery Constraint/4("BattPwrChrgLmt ")
  VehSpd/1 -> Veh2WhlSpd/1
  WhlTrqMaxVec/1 -> Selector2/1, Selector3/1
  WhlEMTrqSplitVecFrnt/1 -> Wheel Torque Vector Logic/2(WhlEMTrqSplitVecFrnt)
  WhlEMTrqSplitVecRear/1 -> Wheel Torque Vector Logic/3(WhlEMTrqSplitVecRear)
  Wheel Torque Vector Logic/2(WhlEMTrqSplitVecRear1) -> EM Constraint Rear/3(WhlEMTrqSplitVecRear)  "WhlEMTrqSplitVecRear"
  [WhlEMTrqSatVecRear] -> Unit Delay/1
  [WhlEMTrqSatVecFrnt] -> Unit Delay1/1
  Unit Delay/1 -> Wheel Torque Vector Logic/4(WhlEMTrqSatVecRear)
  Unit Delay1/1 -> Wheel Torque Vector Logic/5(WhlEMTrqSatVecFrnt)

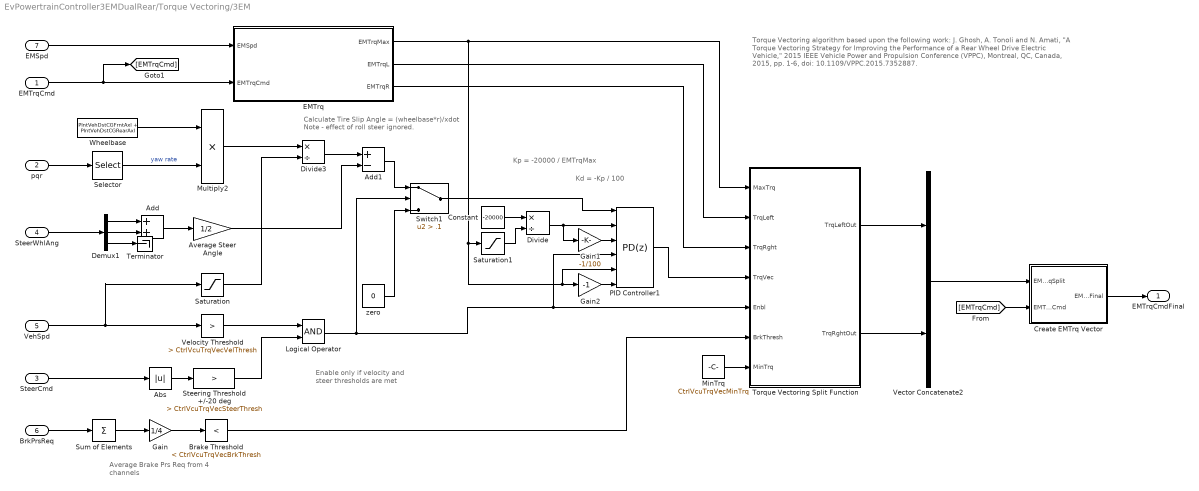
== system EvPowertrainController3EMDualRear/Torque Vectoring/3EM ==
  note: Torque Vectoring algorithm based upon the following work:
      |
      | J. Ghosh, A. Tonoli and N. Amati, "A Torque Vectoring Strategy for Improving the Performance of a Rear Wheel Drive Electric Vehicle," 2015 IEEE Vehicle Power and Propulsion Conference (VPPC), Montreal, QC, Canada, 2015, pp. 1-6, doi: 10.1109/VPPC.2015.7352887.
  note: Kd = -Kp / 100
  note: Kp = -20000 / EMTrqMax
  note: Calculate Tire Slip Angle = (wheelbase*r)/xdot
      | Note - effect of roll steer ignored.
  note: Enable only if velocity and
      | steer thresholds are met
  note: Average Brake Prs Req
      | from 4 channels
  EMTrqCmd : Inport
  pqr : Inport  Port=2
  SteerCmd : Inport  Port=3
  SteerWhlAng : Inport  Port=4
  VehSpd : Inport  Port=5
  BrkPrsReq : Inport  Port=6
  EMSpd : Inport  Port=7
  Abs : Abs  SaturateOnIntegerOverflow=off
  Add : Sum
  Add1 : Sum  Inputs=+-
  Average Steer Angle : Gain  Gain=1/2
  Brake Threshold : simulink/Logic and Bit Operations/Compare To Constant  relop=<  const=CtrlVcuTrqVecBrkThresh  OutDataTypeStr=boolean
  Constant : Constant  Value=-20000  SampleTime=-1
  Create EMTrq Vector : Subsystem  Variant=on  VariantControlMode=label  VariantControl=Choice  LabelModeActiveChoice=3EMDualRear
  Demux1 : Demux  Outputs=[1 1 2]
  Divide : Product  Inputs=*/
  Divide3 : Product  Inputs=*/
  EMTrq : Subsystem  Variant=on  VariantControlMode=label  VariantControl=Choice  LabelModeActiveChoice=3EMDualRear
  Gain : Gain  Gain=1/4
  Gain1 : Gain  Gain=-1/100
  Gain2 : Gain  Gain=-1
  Logical Operator : Logic  AllPortsSameDT=off  OutDataTypeStr=boolean
  MinTrq : Constant  Value=CtrlVcuTrqVecMinTrq  SampleTime=-1
  Multiply2 : Product
  PID Controller1 : slpidlib/PID Controller  Controller=PD  Form=Parallel  TimeDomain=Discrete-time  UseExternalTs=off  SampleTime=-1  IntegratorMethod=Forward Euler  FilterMethod=Forward Euler  ControllerParametersSource=external  P=CtrlVcuTrqVecPGain/10  I=CtrlVcuTrqVecPGain/10  UseKiTs=off  D=0  UseExternalDerivativeSource=off  N=1  UseFilter=off  TunerSelectOption=Transfer Function Based (PID Tuner App)  ZeroCross=off  InitialConditionSource=internal  InitialConditionForIntegrator=0  InitialConditionForFilter=0  DifferentiatorICPrevScaledInput=0  ExternalReset=either  TrackingMode=off  Kt=1  LimitOutput=on  SatLimitsSource=external  UpperSaturationLimit=inf  LowerSaturationLimit=-inf  LinearizeAsGain=on  AntiWindupMode=none  Kb=1  LimitIntegrator=off  UpperIntegratorSaturationLimit=inf  LowerIntegratorSaturationLimit=-inf  POutMin=[]  POutMax=[]  IOutMin=[]  IOutMax=[]  DOutMin=[]  DOutMax=[]  NOutMin=[]  NOutMax=[]  SumOutMin=[]  SumOutMax=[]  SaturationOutMin=[]  SaturationOutMax=[]  PParamMin=[]  PParamMax=[]  IParamMin=[]  IParamMax=[]  DParamMin=[]  DParamMax=[]  NParamMin=[]  NParamMax=[]  KbParamMin=[]  KbParamMax=[]  KtParamMin=[]  KtParamMax=[]  KbOutMin=[]  KbOutMax=[]  KtOutMin=[]  KtOutMax=[]  IntegratorOutMin=[]  IntegratorOutMax=[]  FilterOutMin=[]  FilterOutMax=[]  SumI1OutMin=[]  SumI1OutMax=[]  SumI2OutMin=[]  SumI2OutMax=[]  SumI3OutMin=[]  SumI3OutMax=[]  SumI4OutMin=[]  SumI4OutMax=[]  SumDOutMin=[]  SumDOutMax=[]  DifferentiatorOutMin=[]  DifferentiatorOutMax=[]  FilterDiffOutCoefMin=[]  FilterDiffOutCoefMax=[]  ReciprocalOutMin=[]  ReciprocalOutMax=[]  SumDenOutMin=[]  SumDenOutMax=[]  SumNumOutMin=[]  SumNumOutMax=[]  DivideOutMin=[]  DivideOutMax=[]  UdiffTsProdOutMin=[]  UdiffTsProdOutMax=[]  NTsProdOutMin=[]  NTsProdOutMax=[]  UintegralTsProdOutMin=[]  UintegralTsProdOutMax=[]  UngainTsProdOutMin=[]  UngainTsProdOutMax=[]  ClampingZeroOutDataTypeStr=Inherit: Inherit via back propagation  ClampingZeroOutMin=[]  ClampingZeroOutMax=[]  FilterDenConstantOutDataTypeStr=Inherit: Inherit via back propagation  FilterDenConstantOutMin=[]  FilterDenConstantOutMax=[]  PCopyOutDataTypeStr=Inherit: Inherit via back propagation  PCopyOutMin=[]  PCopyOutMax=[]  NCopyOutDataTypeStr=Inherit: Inherit via back propagation  NCopyOutMin=[]  NCopyOutMax=[]  IntegratorContinuousStateAttributes=''  IntegratorStateMustResolveToSignalObject=off  IntegratorRTWStateStorageClass=Auto  FilterContinuousStateAttributes=''  FilterStateMustResolveToSignalObject=off  FilterRTWStateStorageClass=Auto  ParallelPVariant=ExternalParameters  IdealPVariant=Disabled  IVariant=Disabled  DVariant=ExternalParameters  IntegratorVariant=Disabled  SatVariant=External  AWVariant=Disabled  PCopyVariant=Disabled  TRVariant=Disabled  FdbkBlocksVariant=Forward  IdealPFdbkVariant=Disabled  SatFdbkVariant=Disabled  DerivativeFilterVariant=Differentiator  NVariant=Passthrough  NCopyVariant=Disabled_SignalSpec  FilterICVariant=InternalICsDifferentiator  IntegratorICVariant=Disabled  ExternalResetVariant=ExternalReset  TRSumVariant=Passthrough  SumFdbkVariant=Disabled  SumVariant=Sum_PD  TsampFilterVariant=InternalTs  TsampNgainVariant=Passthrough  TsampIntegralVariant=Disabled_SignalSpec  ExternalSaturationOutDataTypeStr=Inherit: Same as second input  DerivativeSourceVariant=ErrorSignal
  Saturation : Saturate  UpperLimit=inf  LowerLimit=CtrlVcuTrqVecVelThresh
  Saturation1 : Saturate  UpperLimit=inf  LowerLimit=10
  Selector : Selector  InputPortWidth=3  IndexOptions=Index vector (dialog)  Indices=[3]  OutputSizes=1
  Steering Threshold +/-20 deg : simulink/Logic and Bit Operations/Compare To Constant  relop=>  const=CtrlVcuTrqVecSteerThresh  OutDataTypeStr=boolean
  Sum of Elements : Sum  Inputs=+
  Switch1 : Switch  Criteria=u2 > Threshold  Threshold=.1  SaturateOnIntegerOverflow=off  InputSameDT=off
  Terminator : Terminator
  Torque Vectoring Split Function : MATLAB Function  TreatAsAtomicUnit=on
  Vector Concatenate2 : Concatenate
  Velocity Threshold : simulink/Logic and Bit Operations/Compare To Constant  relop=>  const=CtrlVcuTrqVecVelThresh  OutDataTypeStr=boolean
  Wheelbase : Constant  Value=PlntVehDstCGFrntAxl + PlntVehDstCGRearAxl  SampleTime=-1
  zero : Constant  Value=0  SampleTime=-1
  EMTrqCmdFinal : Outport  VectorParamsAs1DForOutWhenUnconnected=off
  wires:
  Selector/1 -> Multiply2/2  "yaw rate"
  Gain/1 -> Brake Threshold/1
  Sum of Elements/1 -> Gain/1
  [EMTrqCmd] -> Create EMTrq Vector/2(EMTrqCmd)
  Vector Concatenate2/1 -> Create EMTrq Vector/1(EMTrqSplit)
  EMTrq/3(EMTrqR) -> Torque Vectoring Split Function/3(TrqRght)
  EMTrq/2(EMTrqL) -> Torque Vectoring Split Function/2(TrqLeft)
  EMSpd/1 -> EMTrq/1(EMSpd)
  Add1/1 -> Switch1/1
  SteerWhlAng/1 -> Demux1/1
  pqr/1 -> Selector/1
  zero/1 -> Switch1/3
  Demux1/1 -> Add/1
  Velocity Threshold/1 -> Logical Operator/1
  Abs/1 -> Steering Threshold +/-20 deg/1
  Torque Vectoring Split Function/1(TrqLeftOut) -> Vector Concatenate2/1
  Steering Threshold +/-20 deg/1 -> Logical Operator/2
  Add/1 -> Average Steer Angle/1
  Torque Vectoring Split Function/2(TrqRghtOut) -> Vector Concatenate2/2
  Brake Threshold/1 -> Torque Vectoring Split Function/6(BrkThresh)
  PID Controller1/1 -> Torque Vectoring Split Function/4(TrqVec)
  Average Steer Angle/1 -> Add1/2
  Multiply2/1 -> Divide3/1
  VehSpd/1 -> Saturation/1, Velocity Threshold/1
  Demux1/2 -> Add/2
  SteerCmd/1 -> Abs/1
  Switch1/1 -> PID Controller1/1
  Divide3/1 -> Add1/1
  BrkPrsReq/1 -> Sum of Elements/1
  Demux1/3 -> Terminator/1
  Wheelbase/1 -> Multiply2/1
  MinTrq/1 -> Torque Vectoring Split Function/7(MinTrq)
  Create EMTrq Vector/1(EMTrqCmdFinal) -> EMTrqCmdFinal/1
  EMTrqCmd/1 -> EMTrq/2(EMTrqCmd), [EMTrqCmd]
  Divide/1 -> Gain1/1, PID Controller1/2
  Gain1/1 -> PID Controller1/3
  Constant/1 -> Divide/1
  EMTrq/1(EMTrqMax) -> Saturation1/1, Gain2/1, PID Controller1/5, Torque Vectoring Split Function/1(MaxTrq)
  Logical Operator/1 -> Switch1/2, Torque Vectoring Split Function/5(Enbl), PID Controller1/4
  Saturation/1 -> Divide3/2
  Gain2/1 -> PID Controller1/6
  Saturation1/1 -> Divide/2

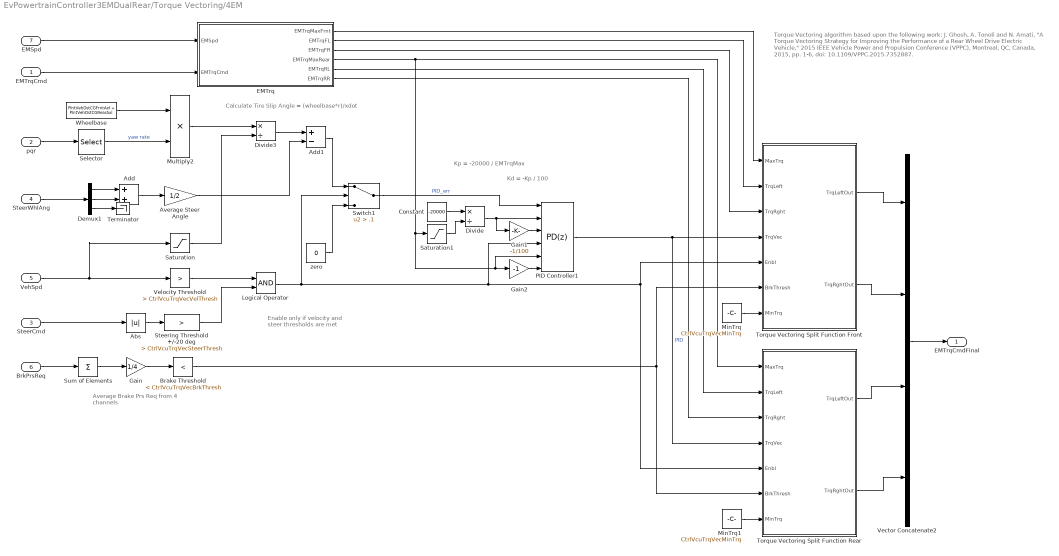
== system EvPowertrainController3EMDualRear/Torque Vectoring/4EM ==
  note: Average Brake Prs Req
      | from 4 channels
  note: Enable only if velocity and
      | steer thresholds are met
  note: Calculate Tire Slip Angle = (wheelbase*r)/xdot
  note: Kd = -Kp / 100
  note: Kp = -20000 / EMTrqMax
  note: Torque Vectoring algorithm based upon the following work:
      |
      | J. Ghosh, A. Tonoli and N. Amati, "A Torque Vectoring Strategy for Improving the Performance of a Rear Wheel Drive Electric Vehicle," 2015 IEEE Vehicle Power and Propulsion Conference (VPPC), Montreal, QC, Canada, 2015, pp. 1-6, doi: 10.1109/VPPC.2015.7352887.
  EMTrqCmd : Inport
  pqr : Inport  Port=2
  SteerCmd : Inport  Port=3
  SteerWhlAng : Inport  Port=4
  VehSpd : Inport  Port=5
  BrkPrsReq : Inport  Port=6
  EMSpd : Inport  Port=7
  Abs : Abs  SaturateOnIntegerOverflow=off
  Add : Sum
  Add1 : Sum  Inputs=+-
  Average Steer Angle : Gain  Gain=1/2
  Brake Threshold : simulink/Logic and Bit Operations/Compare To Constant  relop=<  const=CtrlVcuTrqVecBrkThresh  OutDataTypeStr=boolean
  Constant : Constant  Value=-20000  SampleTime=-1
  Demux1 : Demux  Outputs=[1 1 2]
  Divide : Product  Inputs=*/
  Divide3 : Product  Inputs=*/
  EMTrq : Subsystem
  Gain : Gain  Gain=1/4
  Gain1 : Gain  Gain=-1/100
  Gain2 : Gain  Gain=-1
  Logical Operator : Logic  AllPortsSameDT=off  OutDataTypeStr=boolean
  MinTrq : Constant  Value=CtrlVcuTrqVecMinTrq  SampleTime=-1
  MinTrq1 : Constant  Value=CtrlVcuTrqVecMinTrq  SampleTime=-1
  Multiply2 : Product
  PID Controller1 : slpidlib/PID Controller  Controller=PD  Form=Parallel  TimeDomain=Discrete-time  UseExternalTs=off  SampleTime=-1  IntegratorMethod=Forward Euler  FilterMethod=Forward Euler  ControllerParametersSource=external  P=CtrlVcuTrqVecPGain/10  I=CtrlVcuTrqVecPGain/10  UseKiTs=off  D=0  UseExternalDerivativeSource=off  N=1  UseFilter=off  TunerSelectOption=Transfer Function Based (PID Tuner App)  ZeroCross=off  InitialConditionSource=internal  InitialConditionForIntegrator=0  InitialConditionForFilter=0  DifferentiatorICPrevScaledInput=0  ExternalReset=either  TrackingMode=off  Kt=1  LimitOutput=on  SatLimitsSource=external  UpperSaturationLimit=inf  LowerSaturationLimit=-inf  LinearizeAsGain=on  AntiWindupMode=none  Kb=1  LimitIntegrator=off  UpperIntegratorSaturationLimit=inf  LowerIntegratorSaturationLimit=-inf  POutMin=[]  POutMax=[]  IOutMin=[]  IOutMax=[]  DOutMin=[]  DOutMax=[]  NOutMin=[]  NOutMax=[]  SumOutMin=[]  SumOutMax=[]  SaturationOutMin=[]  SaturationOutMax=[]  PParamMin=[]  PParamMax=[]  IParamMin=[]  IParamMax=[]  DParamMin=[]  DParamMax=[]  NParamMin=[]  NParamMax=[]  KbParamMin=[]  KbParamMax=[]  KtParamMin=[]  KtParamMax=[]  KbOutMin=[]  KbOutMax=[]  KtOutMin=[]  KtOutMax=[]  IntegratorOutMin=[]  IntegratorOutMax=[]  FilterOutMin=[]  FilterOutMax=[]  SumI1OutMin=[]  SumI1OutMax=[]  SumI2OutMin=[]  SumI2OutMax=[]  SumI3OutMin=[]  SumI3OutMax=[]  SumI4OutMin=[]  SumI4OutMax=[]  SumDOutMin=[]  SumDOutMax=[]  DifferentiatorOutMin=[]  DifferentiatorOutMax=[]  FilterDiffOutCoefMin=[]  FilterDiffOutCoefMax=[]  ReciprocalOutMin=[]  ReciprocalOutMax=[]  SumDenOutMin=[]  SumDenOutMax=[]  SumNumOutMin=[]  SumNumOutMax=[]  DivideOutMin=[]  DivideOutMax=[]  UdiffTsProdOutMin=[]  UdiffTsProdOutMax=[]  NTsProdOutMin=[]  NTsProdOutMax=[]  UintegralTsProdOutMin=[]  UintegralTsProdOutMax=[]  UngainTsProdOutMin=[]  UngainTsProdOutMax=[]  ClampingZeroOutDataTypeStr=Inherit: Inherit via back propagation  ClampingZeroOutMin=[]  ClampingZeroOutMax=[]  FilterDenConstantOutDataTypeStr=Inherit: Inherit via back propagation  FilterDenConstantOutMin=[]  FilterDenConstantOutMax=[]  PCopyOutDataTypeStr=Inherit: Inherit via back propagation  PCopyOutMin=[]  PCopyOutMax=[]  NCopyOutDataTypeStr=Inherit: Inherit via back propagation  NCopyOutMin=[]  NCopyOutMax=[]  IntegratorContinuousStateAttributes=''  IntegratorStateMustResolveToSignalObject=off  IntegratorRTWStateStorageClass=Auto  FilterContinuousStateAttributes=''  FilterStateMustResolveToSignalObject=off  FilterRTWStateStorageClass=Auto  ParallelPVariant=ExternalParameters  IdealPVariant=Disabled  IVariant=Disabled  DVariant=ExternalParameters  IntegratorVariant=Disabled  SatVariant=External  AWVariant=Disabled  PCopyVariant=Disabled  TRVariant=Disabled  FdbkBlocksVariant=Forward  IdealPFdbkVariant=Disabled  SatFdbkVariant=Disabled  DerivativeFilterVariant=Differentiator  NVariant=Passthrough  NCopyVariant=Disabled_SignalSpec  FilterICVariant=InternalICsDifferentiator  IntegratorICVariant=Disabled  ExternalResetVariant=ExternalReset  TRSumVariant=Passthrough  SumFdbkVariant=Disabled  SumVariant=Sum_PD  TsampFilterVariant=InternalTs  TsampNgainVariant=Passthrough  TsampIntegralVariant=Disabled_SignalSpec  ExternalSaturationOutDataTypeStr=Inherit: Same as second input  DerivativeSourceVariant=ErrorSignal
  Saturation : Saturate  UpperLimit=inf  LowerLimit=CtrlVcuTrqVecVelThresh
  Saturation1 : Saturate  UpperLimit=inf  LowerLimit=10
  Selector : Selector  InputPortWidth=3  IndexOptions=Index vector (dialog)  Indices=[3]  OutputSizes=1
  Steering Threshold +/-20 deg : simulink/Logic and Bit Operations/Compare To Constant  relop=>  const=CtrlVcuTrqVecSteerThresh  OutDataTypeStr=boolean
  Sum of Elements : Sum  Inputs=+
  Switch1 : Switch  Criteria=u2 > Threshold  Threshold=.1  SaturateOnIntegerOverflow=off  InputSameDT=off
  Terminator : Terminator
  Torque Vectoring Split Function Front : MATLAB Function  TreatAsAtomicUnit=on
  Torque Vectoring Split Function Rear : MATLAB Function  TreatAsAtomicUnit=on
  Vector Concatenate2 : Concatenate  NumInputs=4
  Velocity Threshold : simulink/Logic and Bit Operations/Compare To Constant  relop=>  const=CtrlVcuTrqVecVelThresh  OutDataTypeStr=boolean
  Wheelbase : Constant  Value=PlntVehDstCGFrntAxl + PlntVehDstCGRearAxl  SampleTime=-1
  zero : Constant  Value=0  SampleTime=-1
  EMTrqCmdFinal : Outport  VectorParamsAs1DForOutWhenUnconnected=off
  wires:
  EMTrqCmd/1 -> EMTrq/2(EMTrqCmd)
  Vector Concatenate2/1 -> EMTrqCmdFinal/1
  MinTrq/1 -> Torque Vectoring Split Function Front/7(MinTrq)
  Wheelbase/1 -> Multiply2/1
  Demux1/3 -> Terminator/1
  BrkPrsReq/1 -> Sum of Elements/1
  Divide3/1 -> Add1/1
  Switch1/1 -> PID Controller1/1  "PID_err"
  SteerCmd/1 -> Abs/1
  Demux1/2 -> Add/2
  VehSpd/1 -> Velocity Threshold/1, Saturation/1
  Multiply2/1 -> Divide3/1
  Average Steer Angle/1 -> Add1/2
  PID Controller1/1 -> Torque Vectoring Split Function Rear/4(TrqVec), Torque Vectoring Split Function Front/4(TrqVec)  "PID"
  Brake Threshold/1 -> Torque Vectoring Split Function Rear/6(BrkThresh), Torque Vectoring Split Function Front/6(BrkThresh)
  Torque Vectoring Split Function Front/2(TrqRghtOut) -> Vector Concatenate2/2
  Add/1 -> Average Steer Angle/1
  Steering Threshold +/-20 deg/1 -> Logical Operator/2
  Torque Vectoring Split Function Front/1(TrqLeftOut) -> Vector Concatenate2/1
  Abs/1 -> Steering Threshold +/-20 deg/1
  Velocity Threshold/1 -> Logical Operator/1
  Demux1/1 -> Add/1
  zero/1 -> Switch1/3
  pqr/1 -> Selector/1
  SteerWhlAng/1 -> Demux1/1
  Add1/1 -> Switch1/1
  EMSpd/1 -> EMTrq/1(EMSpd)
  EMTrq/1(EMTrqMaxFrnt) -> Torque Vectoring Split Function Front/1(MaxTrq)
  EMTrq/2(EMTrqFL) -> Torque Vectoring Split Function Front/2(TrqLeft)
  EMTrq/3(EMTrqFR) -> Torque Vectoring Split Function Front/3(TrqRght)
  Sum of Elements/1 -> Gain/1
  Gain/1 -> Brake Threshold/1
  Selector/1 -> Multiply2/2  "yaw rate"
  MinTrq1/1 -> Torque Vectoring Split Function Rear/7(MinTrq)
  EMTrq/5(EMTrqRL) -> Torque Vectoring Split Function Rear/2(TrqLeft)
  EMTrq/6(EMTrqRR) -> Torque Vectoring Split Function Rear/3(TrqRght)
  Torque Vectoring Split Function Rear/1(TrqLeftOut) -> Vector Concatenate2/3
  Torque Vectoring Split Function Rear/2(TrqRghtOut) -> Vector Concatenate2/4
  Gain2/1 -> PID Controller1/6
  Logical Operator/1 -> PID Controller1/4, Torque Vectoring Split Function Rear/5(Enbl), Torque Vectoring Split Function Front/5(Enbl), Switch1/2
  Constant/1 -> Divide/1
  Gain1/1 -> PID Controller1/3
  EMTrq/4(EMTrqMaxRear) -> Saturation1/1, Gain2/1, PID Controller1/5, Torque Vectoring Split Function Rear/1(MaxTrq)
  Divide/1 -> Gain1/1, PID Controller1/2
  Saturation1/1 -> Divide/2
  Saturation/1 -> Divide3/2

== system EvPowertrainController3EMDualRear/Torque Vectoring/No Torque Vectoring ==
  EMTrqCmd : Inport
  EMTrqCmdFinal : Outport  VectorParamsAs1DForOutWhenUnconnected=off
  wires:
  EMTrqCmd/1 -> EMTrqCmdFinal/1

== system EvPowertrainController3EMDualRear/Accel Pedal to Traction Wheel Torque Request/EM2WhlTrq/2EM ==
  note: Reflect EMTrq to WhlTrq
      | due to possible gearing
      | differences
  note: Use VehSpd instead of EMSpd or
      | WhlSpd in case wheel or EM are
      | undergoing slipping / have oscillations.
  Gear : Inport
  VehSpd : Inport  Port=2
  Add : Sum
  EMTrq2WhlTrqFrnt : Subsystem  Variant=on  VariantControlMode=label  VariantControl=1  LabelModeActiveChoice=3
  EMTrq2WhlTrqRear : Subsystem  Variant=on  VariantControlMode=label  VariantControl=1  LabelModeActiveChoice=3
  Maximum Torque Front Axle : Subsystem
  Maximum Torque Rear Axle : Subsystem
  VehSpd2EMSpd : Subsystem  Variant=on  VariantControlMode=label  VariantControl=1  LabelModeActiveChoice=3
  WhlTrqCmd : Outport
  wires:
  Maximum Torque Front Axle/1(EMTrq) -> EMTrq2WhlTrqFrnt/2(EMTrqCmd)
  VehSpd2EMSpd/1(EMSpdFrntAxl) -> EMTrq2WhlTrqFrnt/3(EMSpd), Maximum Torque Front Axle/1(EMSpd)
  Maximum Torque Rear Axle/1(EMTrq) -> EMTrq2WhlTrqRear/2(EMTrqCmd)
  Gear/1 -> VehSpd2EMSpd/1(Gear), EMTrq2WhlTrqFrnt/1(Gear), EMTrq2WhlTrqRear/1(Gear)
  EMTrq2WhlTrqFrnt/1(WhlMotTrq) -> Add/1
  VehSpd/1 -> VehSpd2EMSpd/2(VehSpd)
  Add/1 -> WhlTrqCmd/1
  EMTrq2WhlTrqRear/1(WhlMotTrq) -> Add/2
  VehSpd2EMSpd/2(EMSpdRearAxl) -> EMTrq2WhlTrqRear/3(EMSpd), Maximum Torque Rear Axle/1(EMSpd)

== system EvPowertrainController3EMDualRear/Accel Pedal to Traction Wheel Torque Request/EM2WhlTrq/3EM Dual Front ==
  note: Use VehSpd instead of EMSpd or
      | WhlSpd in case wheel or EM are
      | undergoing slipping / have oscillations.
  note: Reflect EMTrq to WhlTrq
      | due to possible gearing
      | differences
  Gear : Inport
  VehSpd : Inport  Port=2
  Add : Sum
  EMTrq2WhlTrqFrnt : Subsystem  Variant=on  VariantControlMode=label  VariantControl=1  LabelModeActiveChoice=3
  EMTrq2WhlTrqRear : Subsystem  Variant=on  VariantControlMode=label  VariantControl=1  LabelModeActiveChoice=3
  Maximum Torque Front Axle : Subsystem
  Maximum Torque Rear Axle : Subsystem
  VehSpd2EMSpd : Subsystem  Variant=on  VariantControlMode=label  VariantControl=1  LabelModeActiveChoice=3
  WhlTrqCmd : Outport
  wires:
  VehSpd2EMSpd/2(EMSpdRearAxl) -> Maximum Torque Rear Axle/1(EMSpd), EMTrq2WhlTrqRear/3(EMSpd)
  EMTrq2WhlTrqRear/1(WhlMotTrq) -> Add/2
  Add/1 -> WhlTrqCmd/1
  VehSpd/1 -> VehSpd2EMSpd/2(VehSpd)
  EMTrq2WhlTrqFrnt/1(WhlMotTrq) -> Add/1
  Gear/1 -> EMTrq2WhlTrqRear/1(Gear), EMTrq2WhlTrqFrnt/1(Gear), VehSpd2EMSpd/1(Gear)
  Maximum Torque Rear Axle/1(EMTrq) -> EMTrq2WhlTrqRear/2(EMTrqCmd)
  VehSpd2EMSpd/1(EMSpdFrntAxl) -> Maximum Torque Front Axle/1(EMSpd), EMTrq2WhlTrqFrnt/3(EMSpd)
  Maximum Torque Front Axle/1(EMTrq) -> EMTrq2WhlTrqFrnt/2(EMTrqCmd)

== system EvPowertrainController3EMDualRear/Accel Pedal to Traction Wheel Torque Request/EM2WhlTrq/3EM Dual Rear ==
  note: Reflect EMTrq to WhlTrq
      | due to possible gearing
      | differences
  note: Use VehSpd instead of EMSpd or
      | WhlSpd in case wheel or EM are
      | undergoing slipping / have oscillations.
  Gear : Inport
  VehSpd : Inport  Port=2
  Add : Sum
  EMTrq2WhlTrqFrnt : Subsystem  Variant=on  VariantControlMode=label  VariantControl=1  LabelModeActiveChoice=3
  EMTrq2WhlTrqRear : Subsystem  Variant=on  VariantControlMode=label  VariantControl=1  LabelModeActiveChoice=3
  Maximum Torque Front Axle : Subsystem
  Maximum Torque Rear Axle : Subsystem
  VehSpd2EMSpd : Subsystem  Variant=on  VariantControlMode=label  VariantControl=1  LabelModeActiveChoice=3
  WhlTrqCmd : Outport
  wires:
  Maximum Torque Front Axle/1(EMTrq) -> EMTrq2WhlTrqFrnt/2(EMTrqCmd)
  VehSpd2EMSpd/1(EMSpdFrntAxl) -> EMTrq2WhlTrqFrnt/3(EMSpd), Maximum Torque Front Axle/1(EMSpd)
  Maximum Torque Rear Axle/1(EMTrq) -> EMTrq2WhlTrqRear/2(EMTrqCmd)
  Gear/1 -> VehSpd2EMSpd/1(Gear), EMTrq2WhlTrqFrnt/1(Gear), EMTrq2WhlTrqRear/1(Gear)
  EMTrq2WhlTrqFrnt/1(WhlMotTrq) -> Add/1
  VehSpd/1 -> VehSpd2EMSpd/2(VehSpd)
  Add/1 -> WhlTrqCmd/1
  EMTrq2WhlTrqRear/1(WhlMotTrq) -> Add/2
  VehSpd2EMSpd/2(EMSpdRearAxl) -> EMTrq2WhlTrqRear/3(EMSpd), Maximum Torque Rear Axle/1(EMSpd)

== system EvPowertrainController3EMDualRear/Accel Pedal to Traction Wheel Torque Request/EM2WhlTrq/4EM ==
  note: Use VehSpd instead of EMSpd or
      | WhlSpd in case wheel or EM are
      | undergoing slipping / have oscillations.
  note: Reflect EMTrq to WhlTrq
      | due to possible gearing
      | differences
  Gear : Inport
  VehSpd : Inport  Port=2
  Add : Sum
  EMTrq2WhlTrqFrnt : Subsystem  Variant=on  VariantControlMode=label  VariantControl=1  LabelModeActiveChoice=3
  EMTrq2WhlTrqRear : Subsystem  Variant=on  VariantControlMode=label  VariantControl=1  LabelModeActiveChoice=3
  Maximum Torque Front Axle : Subsystem
  Maximum Torque Rear Axle : Subsystem
  VehSpd2EMSpd : Subsystem  Variant=on  VariantControlMode=label  VariantControl=1  LabelModeActiveChoice=3
  WhlTrqCmd : Outport
  wires:
  VehSpd2EMSpd/2(EMSpdRearAxl) -> Maximum Torque Rear Axle/1(EMSpd), EMTrq2WhlTrqRear/3(EMSpd)
  EMTrq2WhlTrqRear/1(WhlMotTrq) -> Add/2
  Add/1 -> WhlTrqCmd/1
  VehSpd/1 -> VehSpd2EMSpd/2(VehSpd)
  EMTrq2WhlTrqFrnt/1(WhlMotTrq) -> Add/1
  Gear/1 -> EMTrq2WhlTrqRear/1(Gear), EMTrq2WhlTrqFrnt/1(Gear), VehSpd2EMSpd/1(Gear)
  Maximum Torque Rear Axle/1(EMTrq) -> EMTrq2WhlTrqRear/2(EMTrqCmd)
  VehSpd2EMSpd/1(EMSpdFrntAxl) -> Maximum Torque Front Axle/1(EMSpd), EMTrq2WhlTrqFrnt/3(EMSpd)
  Maximum Torque Front Axle/1(EMTrq) -> EMTrq2WhlTrqFrnt/2(EMTrqCmd)

== system EvPowertrainController3EMDualRear/Energy Management/Calculate Average EMSpd and Wheel Torque Curves for Front and Rear Axles/2EM ==
  note: Reflect EMTrq to WhlTrq
      | due to possible gearing
      | differences
  EMSpd : Inport
  Gear : Inport  Port=2
  EMTrq2WhlTrqFrnt : Subsystem  Variant=on  VariantControlMode=label  VariantControl=1  LabelModeActiveChoice=3
  EMTrq2WhlTrqRear : Subsystem  Variant=on  VariantControlMode=label  VariantControl=1  LabelModeActiveChoice=3
  Maximum Torque Front Axle : Subsystem
  Maximum Torque Rear Axle : Subsystem
  Selector : Selector  InputPortWidth=2  IndexOptions=Index vector (dialog)  Indices=[1]  OutputSizes=1
  Selector1 : Selector  InputPortWidth=2  IndexOptions=Index vector (dialog)  Indices=[2]  OutputSizes=1
  Vector Concatenate : Concatenate
  Vector Concatenate1 : Concatenate
  EMAvgSpdVec : Outport
  WhlTrqMaxVec : Outport  Port=2
  wires:
  EMSpd/1 -> Selector/1, Selector1/1
  Selector1/1 -> Vector Concatenate1/2, EMTrq2WhlTrqRear/3(EMSpd), Maximum Torque Rear Axle/1(EMSpd)
  EMTrq2WhlTrqRear/1(WhlMotTrq) -> Vector Concatenate/2
  Gear/1 -> EMTrq2WhlTrqFrnt/1(Gear), EMTrq2WhlTrqRear/1(Gear)
  Selector/1 -> Vector Concatenate1/1, EMTrq2WhlTrqFrnt/3(EMSpd), Maximum Torque Front Axle/1(EMSpd)
  EMTrq2WhlTrqFrnt/1(WhlMotTrq) -> Vector Concatenate/1
  Maximum Torque Rear Axle/1(EMTrq) -> EMTrq2WhlTrqRear/2(EMTrqCmd)
  Maximum Torque Front Axle/1(EMTrq) -> EMTrq2WhlTrqFrnt/2(EMTrqCmd)
  Vector Concatenate/1 -> WhlTrqMaxVec/1
  Vector Concatenate1/1 -> EMAvgSpdVec/1
